simulink model "main_improved"  (R2023b)
settings: Solver=ode4  StartTime=t_min_simu  StopTime=t_max_simu  FixedStep=t_step_simu  RelTol=1e-3
undefined symbols (not defined in the file): M
settings Model: Creator=joao_  LastModifiedBy=joao_

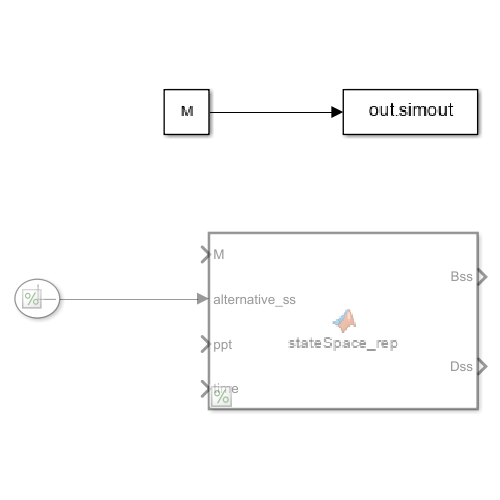
[thumbnail: Simulink's stored preview of the top-level diagram]
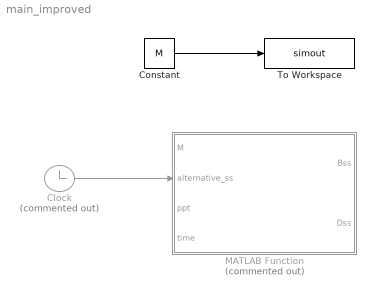
== system main_improved ==
  Clock : Clock  Commented=on
      settings: Decimation=dT_simu
  Constant : Constant  Value=M  VectorParams1D=off
  MATLAB Function : MATLAB Function  Commented=on  TreatAsAtomicUnit=on
  To Workspace : ToWorkspace  VariableName=simout  SaveFormat=Timeseries  SampleTime=-1
  wires:
  Clock/1 -> MATLAB Function/2(alternative_ss)
  Constant/1 -> To Workspace/1

== matlab function main_improved/MATLAB Function ==
  data: M input; alternative_ss input; Bss output; ppt input; time input; Dss output
function [Bss, Dss] = stateSpace_rep(M, alternative_ss, ppt, time)
% This functions return the matrices of an state-space representation (Ass, Bss, Css, Dss) of a dynamical system with the following EOM:
% [M]{xpp} + [C]{xp} + [K]{x} = [G]{p(t)}
%
%
% INPUTS
% M                 -> Mass matrix (associated with the modes)
% alternative_ss    -> Defines the response vector states, 
%                       'd' is displacement only
%                       'v' is velocity only
%                       'a' is acceleration only
%                       'dv' is displacement and velocity
%                       'da' is displacement and acceleration
%                       'va' is velocity and acceleration
%                       'dva' is displacement, velocity and acceleration
%
% It is important to note that the order of the alternative_ss ('va') is sorted in the function so the response vector is sorted alphabetically.
% OUTPUTS
% Bss               -> State-Space Matrix B
% Dss               -> State-Space Matrix D

%% Previous
n_modes = length(M);
n_Pedestrians = ppt(ppt = time);
G = zeros(n_modes, n_Pedestrians);

% State equation matrices
% x' = Ass*x + Bss*p(t)
Bss = [zeros(n_modes); (M^-1)*G];                                         % Input matrix

% Response equation matrices
% y = Css*x + Dss*p(t)                                               % Css is the output matrix and Dss is the feedthrough matrix
alternative = sort(alternative_ss);

if isequal(alternative,'d')
    Dss = zeros(n_modes, n_Pedstrians);

elseif isequal(alternative,'v')
    Dss = zeros(n_modes, n_Pedestrians);

elseif isequal(alternative,'a')
    Dss = (M^-1)*G;

elseif isequal(alternative,'dv')
    Dss = [zeros(n_modes,n_Pedestrians); zeros(n_modes,n_Pedestrians)];

elseif isequal(alternative,'ad')
    Dss = [zeros(n_modes,n_Pedestrians); (M^-1)*G];

elseif isequal(alternative,'av')
    Dss = [zeros(n_modes,n_Pedestrians); (M^-1)*G];

elseif isequal(alternative,'adv')
    Dss = [zeros(n_modes); zeros(n_modes); (M^-1)*G];
end
